simulink model "lab10_nieliniony_sl"  (R2021b)
settings: Solver=VariableStepAuto  StartTime=0.0  StopTime=150.0  RelTol=1e-3
libraries: simulink x2, slpidlib x1
settings Model: Creator=JaSzw  LastModifiedBy=JaSzw

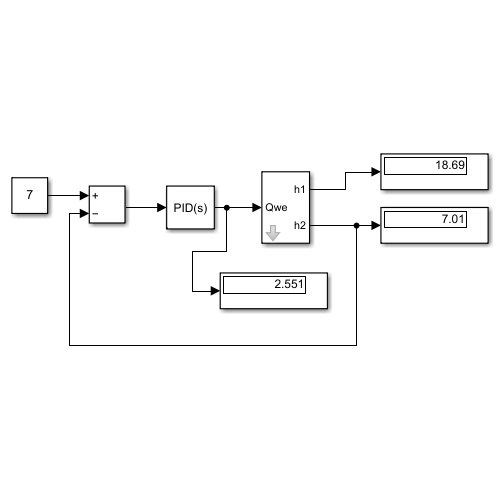
[thumbnail: Simulink's stored preview of the top-level diagram]
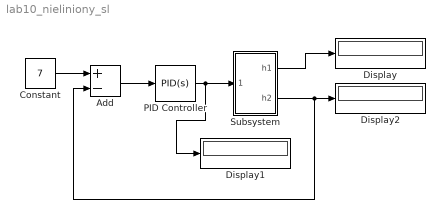
== system lab10_nieliniony_sl ==
  Add : Sum  Inputs=+-
  Constant : Constant  Value=7
  Display : Display
  Display1 : Display
  Display2 : Display
  PID Controller : slpidlib/PID Controller  Controller=PID  Form=Parallel  TimeDomain=Continuous-time  UseExternalTs=off  SampleTime=-1  IntegratorMethod=Forward Euler  FilterMethod=Forward Euler  ControllerParametersSource=internal  P=1  I=0.1  D=0  UseFilter=on  N=100  TunerSelectOption=Transfer Function Based (PID Tuner App)  InitialConditionSource=internal  InitialConditionForIntegrator=0  InitialConditionForFilter=0  DifferentiatorICPrevScaledInput=0  ExternalReset=none  TrackingMode=off  Kt=1  LimitOutput=off  SatLimitsSource=internal  UpperSaturationLimit=inf  LowerSaturationLimit=-inf  LinearizeAsGain=on  AntiWindupMode=none  Kb=1  POutMin=[]  POutMax=[]  IOutMin=[]  IOutMax=[]  DOutMin=[]  DOutMax=[]  NOutMin=[]  NOutMax=[]  SumOutMin=[]  SumOutMax=[]  SaturationOutMin=[]  SaturationOutMax=[]  PParamMin=[]  PParamMax=[]  IParamMin=[]  IParamMax=[]  DParamMin=[]  DParamMax=[]  NParamMin=[]  NParamMax=[]  KbParamMin=[]  KbParamMax=[]  KtParamMin=[]  KtParamMax=[]  KbOutMin=[]  KbOutMax=[]  KtOutMin=[]  KtOutMax=[]  IntegratorOutMin=[]  IntegratorOutMax=[]  FilterOutMin=[]  FilterOutMax=[]  SumI1OutMin=[]  SumI1OutMax=[]  SumI2OutMin=[]  SumI2OutMax=[]  SumI3OutMin=[]  SumI3OutMax=[]  SumI4OutMin=[]  SumI4OutMax=[]  SumDOutMin=[]  SumDOutMax=[]  DifferentiatorOutMin=[]  DifferentiatorOutMax=[]  FilterDiffOutCoefMin=[]  FilterDiffOutCoefMax=[]  ReciprocalOutMin=[]  ReciprocalOutMax=[]  SumDenOutMin=[]  SumDenOutMax=[]  SumNumOutMin=[]  SumNumOutMax=[]  DivideOutMin=[]  DivideOutMax=[]  UdiffTsProdOutMin=[]  UdiffTsProdOutMax=[]  NTsProdOutMin=[]  NTsProdOutMax=[]  UintegralTsProdOutMin=[]  UintegralTsProdOutMax=[]  UngainTsProdOutMin=[]  UngainTsProdOutMax=[]  IntegratorContinuousStateAttributes=''  IntegratorStateMustResolveToSignalObject=off  IntegratorRTWStateStorageClass=Auto  FilterContinuousStateAttributes=''  FilterStateMustResolveToSignalObject=off  FilterRTWStateStorageClass=Auto  ParallelPVariant=InternalParameters  IdealPVariant=Disabled  IVariant=InternalParameters  DVariant=InternalParameters  IntegratorVariant=Continuous  SatVariant=Disabled  AWVariant=Passthrough  PCopyVariant=Disabled  TRVariant=Disabled  FdbkBlocksVariant=Forward  IdealPFdbkVariant=Disabled  SatFdbkVariant=Disabled  DerivativeFilterVariant=ContFilter  NVariant=InternalParameters  NCopyVariant=Disabled  FilterICVariant=InternalICsFilter  IntegratorICVariant=InternalICs  ExternalResetVariant=Disabled  TRSumVariant=Passthrough  SumFdbkVariant=Disabled  SumVariant=Sum_PID  TsampFilterVariant=InternalTs  TsampNgainVariant=Passthrough  TsampIntegralVariant=Passthrough  ExternalSaturationOutDataTypeStr=Inherit: Same as second input
  Subsystem : Subsystem  mask{h1=4, h2=2, S1=1, S2=2, Swy1=0.2, Swy2=0.2, fi1=1, fi2=1, g=9.81, Qwe=2}
  wires:
  PID Controller/1 -> Display1/1, Subsystem/1(Qwe)
  Add/1 -> PID Controller/1
  Constant/1 -> Add/1
  Subsystem/2(h2) -> Add/2, Display2/1
  Subsystem/1(h1) -> Display/1

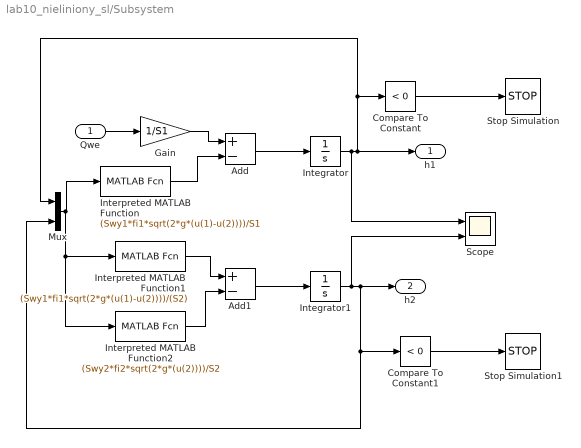
== system lab10_nieliniony_sl/Subsystem ==
  Qwe : Inport
  Add : Sum  Inputs=+-
  Add1 : Sum  Inputs=+-
  Compare To Constant : simulink/Logic and Bit Operations/Compare To Constant  relop=<  const=0  OutDataTypeStr=boolean
  Compare To Constant1 : simulink/Logic and Bit Operations/Compare To Constant  relop=<  const=0  OutDataTypeStr=boolean
  Gain : Gain  Gain=1/S1
  Integrator : Integrator  InitialCondition=h1
  Integrator1 : Integrator  InitialCondition=h2
  Interpreted MATLAB Function : MATLABFcn  MATLABFcn=(Swy1*fi1*sqrt(2*g*(u(1)-u(2))))/S1  OutputDimensions=1
  Interpreted MATLAB Function1 : MATLABFcn  MATLABFcn=(Swy1*fi1*sqrt(2*g*(u(1)-u(2))))/(S2)  OutputDimensions=1
  Interpreted MATLAB Function2 : MATLABFcn  MATLABFcn=(Swy2*fi2*sqrt(2*g*(u(2))))/S2  OutputDimensions=1
  Mux : Mux  Inputs=2
  Scope : Scope  NumInputPorts=2
  Stop Simulation : Stop
  Stop Simulation1 : Stop
  h1 : Outport
  h2 : Outport  Port=2
  wires:
  Integrator/1 -> Scope/1, h1/1, Compare To Constant/1, Mux/1
  Add1/1 -> Integrator1/1
  Add/1 -> Integrator/1
  Interpreted MATLAB Function/1 -> Add/2
  Qwe/1 -> Gain/1
  Mux/1 -> Interpreted MATLAB Function2/1, Interpreted MATLAB Function1/1, Interpreted MATLAB Function/1
  Interpreted MATLAB Function2/1 -> Add1/2
  Interpreted MATLAB Function1/1 -> Add1/1
  Compare To Constant/1 -> Stop Simulation/1
  Integrator1/1 -> Scope/2, h2/1, Compare To Constant1/1, Mux/2
  Compare To Constant1/1 -> Stop Simulation1/1
  Gain/1 -> Add/1
